simulink model "problem_2"  (R2018a)
settings: Solver=VariableStepAuto  StartTime=0.0  StopTime=40  RelTol=1e-3
values from neighbouring files (symbols this model uses):
  A = [0 0 1 0 0 0 0.0009 0 0 ... (first row only)    [model.m]
  B = [0 0 0 ... (first row only)    [model.m]
  C1 = [1 0 0 0 0 0 0 0 0 ... (first row only)    [model.m]
  D_1 = [D1 zeros(9,3) xigma*I1]    [model.m]
  E1 = [E xigma*I1 zeros(9,3)]    [model.m]
  F = -((D_2'*D_2)^-1)*(D_2'*C_2+B'*P)    [model.m]
  K = -(Q*C1'+E1*D_1')*(D_1*D_1')^-1    [model.m]
settings Model: Creator=HP  LastModifiedBy=HP

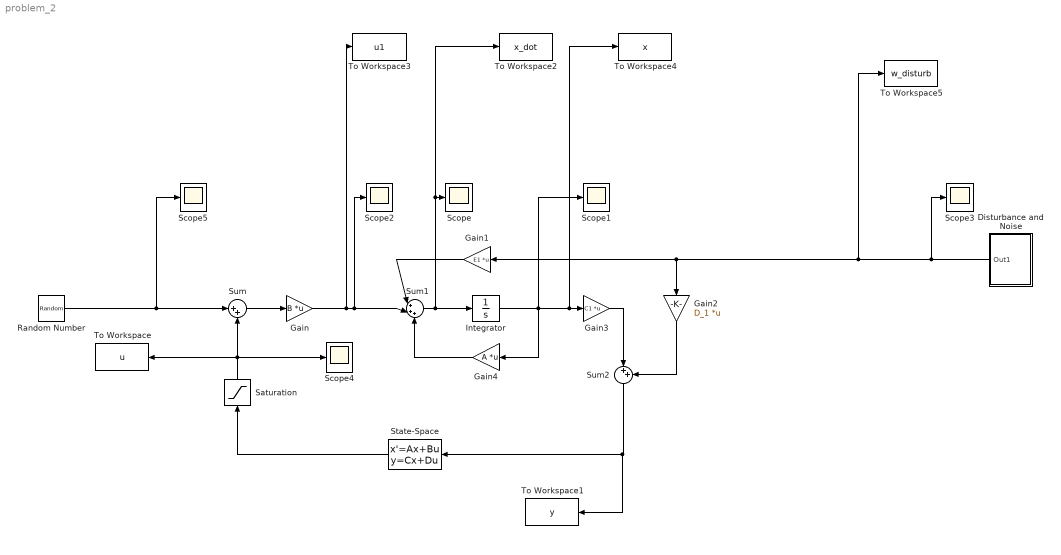
== system problem_2 ==
  Disturbance and Noise : Subsystem
  Gain : Gain  Gain=B  Multiplication=Matrix(K*u) (u vector)
  Gain1 : Gain  Gain=E1  Multiplication=Matrix(K*u) (u vector)
  Gain2 : Gain  Gain=D_1  Multiplication=Matrix(K*u) (u vector)
  Gain3 : Gain  Gain=C1  Multiplication=Matrix(K*u) (u vector)
  Gain4 : Gain  Gain=A  Multiplication=Matrix(K*u) (u vector)
  Integrator : Integrator
  Random Number : RandomNumber  Variance=0.01  SampleTime=0.1  VectorParams1D=off
  Saturation : Saturate  UpperLimit=0.35  LowerLimit=-0.35
  Scope{,1..5} (6 alike) : Scope
  State-Space : StateSpace  A=A+B*F+K*C1  B=-K  C=F  D=zeros(3,9)  InitialCondition=0
  Sum : Sum  Inputs=|++
  Sum1 : Sum  Inputs=|+++
  Sum2 : Sum  Inputs=|++
  To Workspace : ToWorkspace  VariableName=u  SampleTime=-1
  To Workspace1 : ToWorkspace  VariableName=y  SampleTime=-1
  To Workspace2 : ToWorkspace  VariableName=x_dot  SampleTime=-1
  To Workspace3 : ToWorkspace  VariableName=u1  SampleTime=-1
  To Workspace4 : ToWorkspace  VariableName=x  SampleTime=-1
  To Workspace5 : ToWorkspace  VariableName=w_disturb  SampleTime=-1
  wires:
  Sum1/1 -> To Workspace2/1, Scope/1, Integrator/1
  Integrator/1 -> Scope1/1, To Workspace4/1, Gain3/1, Gain4/1
  Gain4/1 -> Sum1/3
  Gain3/1 -> Sum2/1
  Gain2/1 -> Sum2/2
  Gain1/1 -> Sum1/1
  Gain/1 -> Scope2/1, Sum1/2, To Workspace3/1
  Sum/1 -> Gain/1
  Saturation/1 -> Sum/2, Scope4/1, To Workspace/1
  Sum2/1 -> State-Space/1, To Workspace1/1
  Random Number/1 -> Scope5/1, Sum/1
  State-Space/1 -> Saturation/1
  Disturbance and Noise/1(Out1) -> Scope3/1, To Workspace5/1, Gain2/1, Gain1/1

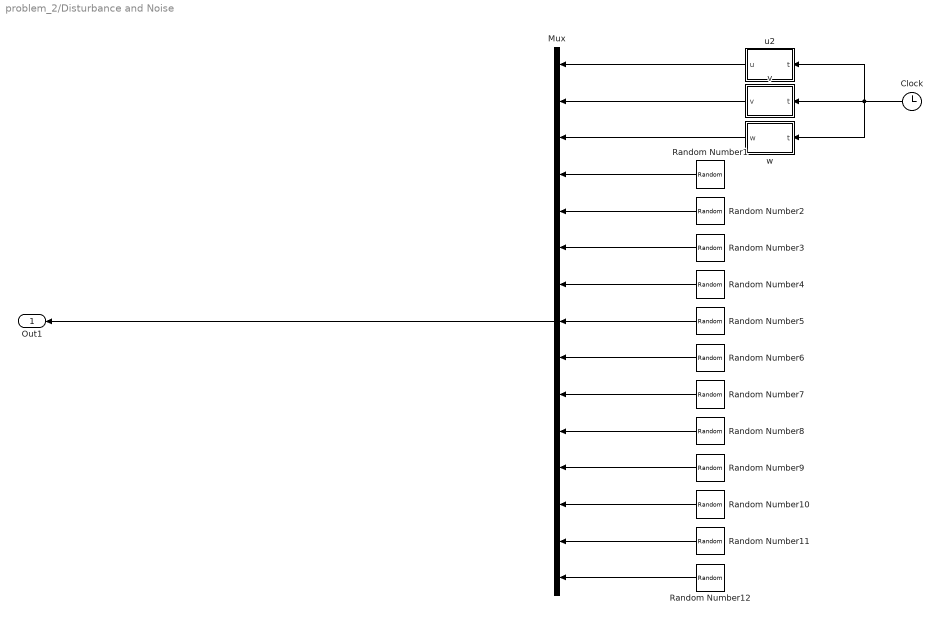
== system problem_2/Disturbance and Noise ==
  Clock : Clock
  Mux : Mux  Inputs=15
  Random Number1 : RandomNumber  Variance=0.01  SampleTime=0.1
  Random Number10 : RandomNumber  Variance=0.01  Seed=9  SampleTime=0.1
  Random Number11 : RandomNumber  Variance=0.01  Seed=10  SampleTime=0.1
  Random Number12 : RandomNumber  Variance=0.01  Seed=11  SampleTime=0.1
  Random Number2 : RandomNumber  Variance=0.01  Seed=1  SampleTime=0.1
  Random Number3 : RandomNumber  Variance=0.01  Seed=2  SampleTime=0.1
  Random Number4 : RandomNumber  Variance=0.01  Seed=3  SampleTime=0.1
  Random Number5 : RandomNumber  Variance=0.01  Seed=4  SampleTime=0.1
  Random Number6 : RandomNumber  Variance=0.01  Seed=5  SampleTime=0.1
  Random Number7 : RandomNumber  Variance=0.01  Seed=6  SampleTime=0.1
  Random Number8 : RandomNumber  Variance=0.01  Seed=7  SampleTime=0.1
  Random Number9 : RandomNumber  Variance=0.01  Seed=8  SampleTime=0.1
  u2 : MATLAB Function  TreatAsAtomicUnit=on
  v : MATLAB Function  TreatAsAtomicUnit=on
  w : MATLAB Function  TreatAsAtomicUnit=on
  Out1 : Outport
  wires:
  v/1(v) -> Mux/2
  Random Number12/1 -> Mux/15
  Random Number8/1 -> Mux/11
  w/1(w) -> Mux/3
  Clock/1 -> u2/1(t), w/1(t), v/1(t)
  Random Number3/1 -> Mux/6
  Random Number6/1 -> Mux/9
  Random Number9/1 -> Mux/12
  Random Number1/1 -> Mux/4
  Random Number10/1 -> Mux/13
  Random Number5/1 -> Mux/8
  Random Number4/1 -> Mux/7
  u2/1(u) -> Mux/1
  Random Number2/1 -> Mux/5
  Random Number7/1 -> Mux/10
  Random Number11/1 -> Mux/14
  Mux/1 -> Out1/1

== matlab function problem_2/Disturbance and Noise/v ==
  data: t input; v output
function v = fcn(t)
if (t>=10&&t<=30)
v =10*cos(2*pi/40*(t-20));
else
    v=0;
end

== matlab function problem_2/Disturbance and Noise/u2 ==
  data: t input; u output
function u = fcn(t)
if (t>=10&&t<=30)
u =10*cos(2*pi/40*(t-20));
else
    u=0;
end

== matlab function problem_2/Disturbance and Noise/w ==
  data: t input; w output
function w = fcn(t)
if (t>=10&&t<=30)
w = 3*cos(2*pi/40*(t-20));
else
    w=0;
end
